simulink library "csu_ctp_coarse_thruster_pulse_command_new_lib"  (R2015b)
settings: Solver=ode113  StartTime=0.0  StopTime=10.0  RelTol=1e-3
values from neighbouring files (symbols this model uses):
  cac_acs_minimum_coarse_thruster_ontime = 30    [csc_cac_coarse_acs_ctrl_init.m]
  cac_acs_time_gain_x = 20.0    (= 20)    [csc_cac_coarse_acs_ctrl_init.m]
  cac_acs_time_gain_y = 20.0    (= 20)    [csc_cac_coarse_acs_ctrl_init.m]
  cac_acs_time_gain_z = 20.0    (= 20)    [csc_cac_coarse_acs_ctrl_init.m]
  cac_coarse_desired_thrust_gain = 1.0    (= 1)    [csc_cac_coarse_acs_ctrl_init.m]
  cac_coarse_thruster_force = psp_coarse_acs_thrust    [csc_cac_coarse_acs_ctrl_prep.m]
  cac_coarse_thruster_trq_x = cac_coarse_thruster_trq_x + cac_coarse_thruster_force*cac_coarse_trq_matx(cac_thruster_alloc_coarse_x_plus(i),1)    [csc_cac_coarse_acs_ctrl_prep.m]
  cac_coarse_thruster_trq_y = cac_coarse_thruster_trq_y + cac_coarse_thruster_force*cac_coarse_trq_matx(cac_thruster_alloc_coarse_y_plus(i),2)    [csc_cac_coarse_acs_ctrl_prep.m]
  cac_coarse_thruster_trq_z = cac_coarse_thruster_trq_z + cac_coarse_thruster_force*cac_coarse_trq_matx(cac_thruster_alloc_coarse_z_plus(i),3)    [csc_cac_coarse_acs_ctrl_prep.m]
  cac_max_thrust_to_weight_ratio = 1.05    [csc_cac_coarse_acs_ctrl_init.m]
  cac_saturation_axial_force = 0*cac_coarse_thruster_force*cosd(15)+4*cac_coarse_thruster_force    [csc_cac_coarse_acs_ctrl_prep.m]
  cac_total_trq_axial_force_matx = [cac_coarse_thruster_force*cac_coarse_trq_matx';cac_coarse_thruster_force_axial]    [csc_cac_coarse_acs_ctrl_prep.m]
undefined symbols (not defined in the file or in its folder): cac_num_variable, cac_thr_control, cac_thruster_alloc_pad_coarse_x_tq_full_on, cac_thruster_alloc_pad_coarse_x_tq_variable, cac_thruster_alloc_pad_coarse_y_tq_full_on, cac_thruster_alloc_pad_coarse_y_tq_variable, cac_trq_control, emp_initial_mass, gal_grav_surface_topo
libraries: simulink x12, util_info_lib x2
(part 2 of 2)

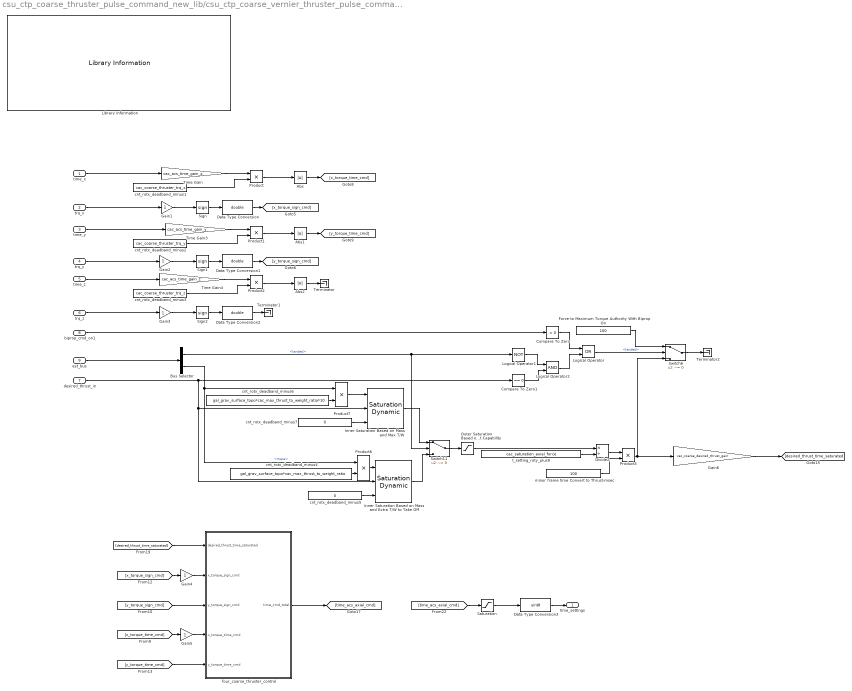
== system csu_ctp_coarse_thruster_pulse_command_new_lib/csu_ctp_coarse_vernier_thruster_pulse_command_new ==
  time_x : Inport
  "trq_x " : Inport  Port=2
  time_y : Inport  Port=3
  trq_y : Inport  Port=4
  time_z : Inport  Port=5
  trq_z : Inport  Port=6
  desired_thrust_in : Inport  Port=7
  biprop_cmd_on1 : Inport  Port=8
  est_bus : Inport  Port=9
  Abs : Abs
  Abs1 : Abs
  Abs2 : Abs
  Bus Selector : BusSelector  OutputSignals=landed,mass
  Compare To Zero : simulink/Logic and Bit Operations/Compare To Zero  relop=>  OutDataTypeStr=boolean
  Compare To Zero1 : simulink/Logic and Bit Operations/Compare To Zero  relop===  OutDataTypeStr=boolean
  Data Type Conversion : DataTypeConversion  OutDataTypeStr=double
  Data Type Conversion1 : DataTypeConversion  OutDataTypeStr=double
  Data Type Conversion2 : DataTypeConversion  OutDataTypeStr=double
  Data Type Conversion3 : DataTypeConversion  OutDataTypeStr=uint8
  Divide2 : Product  Inputs=*/
  Force to Maximum Torque Authority With Biprop On : Constant  Value=100
  Gain{1..5} (5 alike) : Gain
  Gain6 : Gain  Gain=cac_coarse_desired_thrust_gain
  Inner Saturation Based on Mass and Extra T/W to Take Off : simulink/Discontinuities/Saturation Dynamic  OutMin=[]  OutMax=[]  OutDataTypeStr=Inherit: Same as second input  OutDataType=fixdt(1, 16)  OutScaling=2^-10  DoSatur=off
  Inner Saturation Based on Mass and Max T/W : simulink/Discontinuities/Saturation Dynamic  OutMin=[]  OutMax=[]  OutDataTypeStr=Inherit: Same as second input  OutDataType=fixdt(1, 16)  OutScaling=2^-10  DoSatur=off
  Library Information : util_info_lib/Library Information  owner='NONE'
  Logical Operator : Logic  Operator=OR  AllPortsSameDT=off  OutDataTypeStr=boolean
  Logical Operator1 : Logic  Operator=NOT  AllPortsSameDT=off  OutDataTypeStr=boolean
  Logical Operator2 : Logic  AllPortsSameDT=off  OutDataTypeStr=boolean
  Outer Saturation Based on Total Thrust Capability : Saturate  UpperLimit=cac_saturation_axial_force  LowerLimit=0
  Product{,1..3,6..7} (6 alike) : Product
  Saturation : Saturate  UpperLimit=120  LowerLimit=0
  Sign : Signum
  Sign1 : Signum
  Sign2 : Signum
  Switch11 : Switch  Criteria=u2 ~= 0
  Switch6 : Switch  Criteria=u2 ~= 0
  Terminator : Terminator
  Terminator1 : Terminator
  Terminator2 : Terminator
  Time Gain : Gain  Gain=cac_acs_time_gain_x
  Time Gain3 : Gain  Gain=cac_acs_time_gain_y
  Time Gain4 : Gain  Gain=cac_acs_time_gain_z
  cnt_rotx_deadband_minus1 : Constant  Value=cac_coarse_thruster_trq_x
  cnt_rotx_deadband_minus2 : Constant  Value=cac_coarse_thruster_trq_y
  cnt_rotx_deadband_minus3 : Constant  Value=cac_coarse_thruster_trq_z
  cnt_rotx_deadband_minus4 : Constant  Value=gal_grav_surface_topo*cac_max_thrust_to_weight_ratio
  cnt_rotx_deadband_minus5 : Constant  Value=0
  cnt_rotx_deadband_minus6 : Constant  Value=gal_grav_surface_topo*cac_max_thrust_to_weight_ratio*10
  cnt_rotx_deadband_minus7 : Constant  Value=0
  four_coarse_thruster_control : MATLAB Function  TreatAsAtomicUnit=on
  "minor frame time Convert to Thrust-msec " : Constant  Value=100
  t_setting_roty_plus9 : Constant  Value=cac_saturation_axial_force
  time_settings : Outport
  wires:
  Inner Saturation Based on Mass and Max T/W/1 -> Switch11/1
  Product3/1 -> Gain6/1, Switch6/3
  Logical Operator/1 -> Switch6/2  "<landed>"
  desired_thrust_in/1 -> Inner Saturation Based on Mass and Extra T/W to Take Off/2, Inner Saturation Based on Mass and Max T/W/2, Compare To Zero1/1
  Abs1/1 -> [y_torque_time_cmd]
  Abs/1 -> [x_torque_time_cmd]
  Inner Saturation Based on Mass and Extra T/W to Take Off/1 -> Switch11/3
  Time Gain/1 -> Product/1
  Switch11/1 -> Outer Saturation Based on Total Thrust Capability/1
  Bus Selector/1 -> Switch11/2, Logical Operator1/1  "<landed>"
  Logical Operator2/1 -> Logical Operator/2
  Compare To Zero1/1 -> Logical Operator2/2
  Logical Operator1/1 -> Logical Operator2/1
  Compare To Zero/1 -> Logical Operator/1
  Force to Maximum Torque Authority With Biprop On/1 -> Switch6/1
  Outer Saturation Based on Total Thrust Capability/1 -> Divide2/1
  biprop_cmd_on1/1 -> Compare To Zero/1
  four_coarse_thruster_control/1(time_cmd_total) -> [time_acs_axial_cmd]
  Time Gain3/1 -> Product1/1
  [desired_thrust_time_saturated] -> four_coarse_thruster_control/1(desired_thrust_time_saturated)
  Time Gain4/1 -> Product2/1
  [x_torque_sign_cmd] -> Gain4/1
  Abs2/1 -> Terminator/1
  Product2/1 -> Abs2/1
  [x_torque_time_cmd] -> Gain5/1
  [y_torque_sign_cmd] -> four_coarse_thruster_control/3(y_torque_sign_cmd)
  [y_torque_time_cmd] -> four_coarse_thruster_control/5(y_torque_time_cmd)
  Data Type Conversion/1 -> [x_torque_sign_cmd]
  Data Type Conversion1/1 -> [y_torque_sign_cmd]
  Data Type Conversion2/1 -> Terminator1/1
  trq_z/1 -> Gain3/1
  Sign2/1 -> Data Type Conversion2/1
  trq_y/1 -> Gain2/1
  Sign1/1 -> Data Type Conversion1/1
  "trq_x "/1 -> Gain1/1
  Sign/1 -> Data Type Conversion/1
  Divide2/1 -> Product3/1
  t_setting_roty_plus9/1 -> Divide2/2
  "minor frame time Convert to Thrust-msec "/1 -> Product3/2
  Product1/1 -> Abs1/1
  Product/1 -> Abs/1
  cnt_rotx_deadband_minus3/1 -> Product2/2
  cnt_rotx_deadband_minus2/1 -> Product1/2
  time_z/1 -> Time Gain4/1
  time_y/1 -> Time Gain3/1
  time_x/1 -> Time Gain/1
  cnt_rotx_deadband_minus1/1 -> Product/2
  Data Type Conversion3/1 -> time_settings/1
  est_bus/1 -> Bus Selector/1
  cnt_rotx_deadband_minus5/1 -> Inner Saturation Based on Mass and Extra T/W to Take Off/3
  cnt_rotx_deadband_minus4/1 -> Product6/2
  Product6/1 -> Inner Saturation Based on Mass and Extra T/W to Take Off/1
  cnt_rotx_deadband_minus7/1 -> Inner Saturation Based on Mass and Max T/W/3
  cnt_rotx_deadband_minus6/1 -> Product7/2
  Product7/1 -> Inner Saturation Based on Mass and Max T/W/1
  Bus Selector/2 -> Product6/1, Product7/1  "<mass>"
  Gain1/1 -> Sign/1
  Gain2/1 -> Sign1/1
  Gain3/1 -> Sign2/1
  Saturation/1 -> Data Type Conversion3/1
  [time_acs_axial_cmd] -> Saturation/1
  Switch6/1 -> Terminator2/1
  Gain4/1 -> four_coarse_thruster_control/2(x_torque_sign_cmd)
  Gain5/1 -> four_coarse_thruster_control/4(x_torque_time_cmd)
  Gain6/1 -> [desired_thrust_time_saturated]

== matlab function csu_ctp_coarse_thruster_pulse_command_new_lib/csu_ctp_coarse_thruster_pulse_command_short_fire/MATLAB Function ==
  data: x_torque_sign_cmd input; y_torque_sign_cmd input; z_torque_sign_cmd input; x_torque_time_cmd input; y_torque_time_cmd input; z_torque_time_cmd input; x_sorted_thrust_cmd input; y_sorted_thrust_cmd input; desired_thrust_saturated input; cac_trq_control input; cac_thr_control input; cac_thruster_alloc_pad_coarse_x_tq_full_on input; cac_thruster_alloc_pad_coarse_y_tq_full_on input; cac_thruster_alloc_pad_coarse_x_tq_variable input; cac_thruster_alloc_pad_coarse_y_tq_variable input; cac_num_variable input; cac_total_trq_axial_force_matx input; cac_coarse_thruster_trq_x input; cac_coarse_thruster_trq_y input; cac_coarse_thruster_trq_z input; cac_saturation_axial_force input; time_cmd_total output; max_offset_x output; max_offset_y output; dist_thrust_x output; dist_thrust_y output; zone_radius output; radius_minus_distance_x output; radius_minus_distance_y output; imax_x output; imax_y output; delta_thr_x output; delta_thr_y output; delta_trq_x output; delta_trq_y output; coarse_tq_full_on_x output; coarse_tq_full_on_y output; time_axial_cmd output; torq_axial_cmd output; cac_trq_axial_force_pinv_reduced_matx output
function [time_cmd_total,max_offset_x,max_offset_y,...
    dist_thrust_x,dist_thrust_y,...
    zone_radius,...
    radius_minus_distance_x,radius_minus_distance_y,...
    imax_x,imax_y,...
    delta_thr_x,delta_thr_y,...
    delta_trq_x,delta_trq_y,...
    coarse_tq_full_on_x,coarse_tq_full_on_y,...
    time_axial_cmd,torq_axial_cmd,...
    cac_trq_axial_force_pinv_reduced_matx...
     ]...
     =...
                         find_thruster_combination(...
                         x_torque_sign_cmd,...
                         y_torque_sign_cmd,...
                         z_torque_sign_cmd,...
                         x_torque_time_cmd,...
                         y_torque_time_cmd,...
                         z_torque_time_cmd,...
                         x_sorted_thrust_cmd,...
                         y_sorted_thrust_cmd,...
                         desired_thrust_saturated,...
                         cac_trq_control,...
                         cac_thr_control,...
                         cac_thruster_alloc_pad_coarse_x_tq_full_on,...
                         cac_thruster_alloc_pad_coarse_y_tq_full_on,...
                         cac_thruster_alloc_pad_coarse_x_tq_variable,...
                         cac_thruster_alloc_pad_coarse_y_tq_variable,...
                         cac_num_variable,...
                         cac_total_trq_axial_force_matx,...
                         cac_coarse_thruster_trq_x,...
                         cac_coarse_thruster_trq_y,...
                         cac_coarse_thruster_trq_z,...
                         cac_saturation_axial_force...
                         )         
%#codegen

delta_thr_x = zeros(21,1);
delta_thr_y = zeros(21,1);
delta_trq_x = zeros(21,1);
delta_trq_y = zeros(21,1);
dist_thrust_x = zeros(21,1);
dist_thrust_y = zeros(21,1);
zone_radius = zeros(21,1);
radius_minus_distance_x = zeros(21,1);
radius_minus_distance_y = zeros(21,1);
cac_trq_axial_force_reduced_matx = zeros(4,12);

for i=1:size(cac_thr_control,1);
    delta_thr_x(i) = abs(cac_thr_control(i) - x_sorted_thrust_cmd);
    delta_thr_y(i) = abs(cac_thr_control(i) - y_sorted_thrust_cmd);
    
    delta_trq_x(i) = abs(x_torque_sign_cmd*x_torque_time_cmd - cac_trq_control(i));
    delta_trq_y(i) = abs(y_torque_sign_cmd*y_torque_time_cmd - cac_trq_control(i));
    
    dist_thrust_x(i) = sqrt(delta_thr_x(i)^2 + delta_trq_x(i)^2);
    dist_thrust_y(i) = sqrt(delta_thr_y(i)^2 + delta_trq_y(i)^2);
    
    zone_radius(i) = 25 * cac_num_variable(i) * sqrt(2)/2;
    
    radius_minus_distance_x(i) = zone_radius(i) - dist_thrust_x(i);
    radius_minus_distance_y(i) = zone_radius(i) - dist_thrust_y(i);
    
end

[x,imax_x] = max(radius_minus_distance_x);
[y,imax_y] = max(radius_minus_distance_y);
max_offset_x = max(radius_minus_distance_x);
max_offset_y = max(radius_minus_distance_y);

coarse_tq_full_on_x = cac_thruster_alloc_pad_coarse_x_tq_full_on(imax_x,:);
coarse_tq_full_on_y = cac_thruster_alloc_pad_coarse_y_tq_full_on(imax_y,:);

coarse_tq_variable_on_x = cac_thruster_alloc_pad_coarse_x_tq_variable(imax_x,:);
coarse_tq_variable_on_y = cac_thruster_alloc_pad_coarse_y_tq_variable(imax_y,:);

% if max_offset_x <= 0
%     coarse_tq_full_on_x = coarse_tq_full_on_x*0;
%     coarse_tq_variable_on_x = coarse_tq_variable_on_x*0;
% end
% if max_offset_x <= 0
%     coarse_tq_full_on_y = coarse_tq_full_on_y*0;
%     coarse_tq_variable_on_y = coarse_tq_variable_on_y*0;    
% end
% 
for i=1:size(cac_total_trq_axial_force_matx,1)
    cac_trq_axial_force_reduced_matx(i,:) = (cac_total_trq_axial_force_matx(i,:).*(coarse_tq_variable_on_x + coarse_tq_variable_on_y));
end    
cac_trq_axial_force_pinv_reduced_matx = pinv(cac_trq_axial_force_reduced_matx);

time_x_tq_cmd = cac_coarse_thruster_trq_x * x_torque_time_cmd * x_torque_sign_cmd;
time_y_tq_cmd = cac_coarse_thruster_trq_y * y_torque_time_cmd * y_torque_sign_cmd;
time_z_tq_cmd = cac_coarse_thruster_trq_z * z_torque_time_cmd * z_torque_sign_cmd;

time_axial_cmd = 0.0;

if(desired_thrust_saturated > 0.001)
    time_axial_cmd = (x_sorted_thrust_cmd + y_sorted_thrust_cmd)*50;%*desired_thrust_saturated;%*sum(coarse_tq_variable_on_x + coarse_tq_variable_on_y);
end

torq_axial_cmd = [time_x_tq_cmd; time_y_tq_cmd; time_z_tq_cmd ; time_axial_cmd];
time_cmd_total = cac_trq_axial_force_pinv_reduced_matx*torq_axial_cmd + (coarse_tq_full_on_x + coarse_tq_full_on_y)'*100;

== matlab function csu_ctp_coarse_thruster_pulse_command_new_lib/csu_ctp_coarse_thruster_pulse_command_old/MATLAB Function ==
  data: x_torque_sign_cmd input; y_torque_sign_cmd input; z_torque_sign_cmd input; x_torque_time_cmd input; y_torque_time_cmd input; z_torque_time_cmd input; x_sorted_thrust_cmd input; y_sorted_thrust_cmd input; desired_thrust_saturated input; cac_trq_control input; cac_thr_control input; cac_thruster_alloc_pad_coarse_x_tq_full_on input; cac_thruster_alloc_pad_coarse_y_tq_full_on input; cac_thruster_alloc_pad_coarse_x_tq_variable input; cac_thruster_alloc_pad_coarse_y_tq_variable input; cac_num_variable input; cac_total_trq_axial_force_matx input; cac_coarse_thruster_trq_x input; cac_coarse_thruster_trq_y input; cac_coarse_thruster_trq_z input; cac_saturation_axial_force input; time_cmd_total output; max_offset_x output; max_offset_y output; dist_thrust_x output; dist_thrust_y output; zone_radius output; radius_minus_distance_x output; radius_minus_distance_y output; imax_x output; imax_y output; delta_thr_x output; delta_thr_y output; delta_trq_x output; delta_trq_y output; coarse_tq_full_on_x output; coarse_tq_full_on_y output; time_axial_cmd output; torq_axial_cmd output; cac_trq_axial_force_pinv_reduced_matx output
function [time_cmd_total,max_offset_x,max_offset_y,...
    dist_thrust_x,dist_thrust_y,...
    zone_radius,...
    radius_minus_distance_x,radius_minus_distance_y,...
    imax_x,imax_y,...
    delta_thr_x,delta_thr_y,...
    delta_trq_x,delta_trq_y,...
    coarse_tq_full_on_x,coarse_tq_full_on_y,...
    time_axial_cmd,torq_axial_cmd,...
    cac_trq_axial_force_pinv_reduced_matx...
     ]...
     =...
                         find_thruster_combination(...
                         x_torque_sign_cmd,...
                         y_torque_sign_cmd,...
                         z_torque_sign_cmd,...
                         x_torque_time_cmd,...
                         y_torque_time_cmd,...
                         z_torque_time_cmd,...
                         x_sorted_thrust_cmd,...
                         y_sorted_thrust_cmd,...
                         desired_thrust_saturated,...
                         cac_trq_control,...
                         cac_thr_control,...
                         cac_thruster_alloc_pad_coarse_x_tq_full_on,...
                         cac_thruster_alloc_pad_coarse_y_tq_full_on,...
                         cac_thruster_alloc_pad_coarse_x_tq_variable,...
                         cac_thruster_alloc_pad_coarse_y_tq_variable,...
                         cac_num_variable,...
                         cac_total_trq_axial_force_matx,...
                         cac_coarse_thruster_trq_x,...
                         cac_coarse_thruster_trq_y,...
                         cac_coarse_thruster_trq_z,...
                         cac_saturation_axial_force...
                         )         
%#codegen

delta_thr_x = zeros(21,1);
delta_thr_y = zeros(21,1);
delta_trq_x = zeros(21,1);
delta_trq_y = zeros(21,1);
dist_thrust_x = zeros(21,1);
dist_thrust_y = zeros(21,1);
zone_radius = zeros(21,1);
radius_minus_distance_x = zeros(21,1);
radius_minus_distance_y = zeros(21,1);
cac_trq_axial_force_reduced_matx = zeros(4,12);

for i=1:size(cac_thr_control,1);
    delta_thr_x(i) = abs(cac_thr_control(i) - x_sorted_thrust_cmd);
    delta_thr_y(i) = abs(cac_thr_control(i) - y_sorted_thrust_cmd);
    
    delta_trq_x(i) = abs(x_torque_sign_cmd*x_torque_time_cmd - cac_trq_control(i));
    delta_trq_y(i) = abs(y_torque_sign_cmd*y_torque_time_cmd - cac_trq_control(i));
    
    dist_thrust_x(i) = sqrt(delta_thr_x(i)^2 + delta_trq_x(i)^2);
    dist_thrust_y(i) = sqrt(delta_thr_y(i)^2 + delta_trq_y(i)^2);
    
    zone_radius(i) = 25 * cac_num_variable(i) * sqrt(2)/2;
    
    radius_minus_distance_x(i) = zone_radius(i) - dist_thrust_x(i);
    radius_minus_distance_y(i) = zone_radius(i) - dist_thrust_y(i);
    
end

[x,imax_x] = max(radius_minus_distance_x);
[y,imax_y] = max(radius_minus_distance_y);
max_offset_x = max(radius_minus_distance_x);
max_offset_y = max(radius_minus_distance_y);

coarse_tq_full_on_x = cac_thruster_alloc_pad_coarse_x_tq_full_on(imax_x,:);
coarse_tq_full_on_y = cac_thruster_alloc_pad_coarse_y_tq_full_on(imax_y,:);

coarse_tq_variable_on_x = cac_thruster_alloc_pad_coarse_x_tq_variable(imax_x,:);
coarse_tq_variable_on_y = cac_thruster_alloc_pad_coarse_y_tq_variable(imax_y,:);

% if max_offset_x <= 0
%     coarse_tq_full_on_x = coarse_tq_full_on_x*0;
%     coarse_tq_variable_on_x = coarse_tq_variable_on_x*0;
% end
% if max_offset_x <= 0
%     coarse_tq_full_on_y = coarse_tq_full_on_y*0;
%     coarse_tq_variable_on_y = coarse_tq_variable_on_y*0;    
% end
% 
for i=1:size(cac_total_trq_axial_force_matx,1)
    cac_trq_axial_force_reduced_matx(i,:) = (cac_total_trq_axial_force_matx(i,:).*(coarse_tq_variable_on_x + coarse_tq_variable_on_y));
end    
cac_trq_axial_force_pinv_reduced_matx = pinv(cac_trq_axial_force_reduced_matx);

time_x_tq_cmd = cac_coarse_thruster_trq_x * x_torque_time_cmd * x_torque_sign_cmd;
time_y_tq_cmd = cac_coarse_thruster_trq_y * y_torque_time_cmd * y_torque_sign_cmd;
time_z_tq_cmd = cac_coarse_thruster_trq_z * z_torque_time_cmd * z_torque_sign_cmd;

time_axial_cmd = 0.0;

if(desired_thrust_saturated > 0.001)
    time_axial_cmd = (x_sorted_thrust_cmd + y_sorted_thrust_cmd)*50;%*desired_thrust_saturated;%*sum(coarse_tq_variable_on_x + coarse_tq_variable_on_y);
end

torq_axial_cmd = [time_x_tq_cmd; time_y_tq_cmd; time_z_tq_cmd ; time_axial_cmd];
time_cmd_total = cac_trq_axial_force_pinv_reduced_matx*torq_axial_cmd + (coarse_tq_full_on_x + coarse_tq_full_on_y)'*100;

== matlab function csu_ctp_coarse_thruster_pulse_command_new_lib/csu_ctp_coarse_thruster_pulse_command_new/MATLAB Function ==
  data: x_torque_sign_cmd input; y_torque_sign_cmd input; z_torque_sign_cmd input; x_torque_time_cmd input; y_torque_time_cmd input; z_torque_time_cmd input; x_sorted_thrust_cmd input; y_sorted_thrust_cmd input; desired_thrust_saturated input; cac_trq_control input; cac_thr_control input; cac_thruster_alloc_pad_coarse_x_tq_full_on input; cac_thruster_alloc_pad_coarse_y_tq_full_on input; cac_thruster_alloc_pad_coarse_x_tq_variable input; cac_thruster_alloc_pad_coarse_y_tq_variable input; cac_num_variable input; cac_total_trq_axial_force_matx input; cac_coarse_thruster_trq_x input; cac_coarse_thruster_trq_y input; cac_coarse_thruster_trq_z input; cac_saturation_axial_force input; time_cmd_total output; max_offset_x output; max_offset_y output; dist_thrust_x output; dist_thrust_y output; zone_radius output; radius_minus_distance_x output; radius_minus_distance_y output; imax_x output; imax_y output; delta_thr_x output; delta_thr_y output; delta_trq_x output; delta_trq_y output; coarse_tq_full_on_x output; coarse_tq_full_on_y output; time_axial_cmd output; torq_axial_cmd output; cac_trq_axial_force_pinv_reduced_matx output
function [time_cmd_total,max_offset_x,max_offset_y,...
    dist_thrust_x,dist_thrust_y,...
    zone_radius,...
    radius_minus_distance_x,radius_minus_distance_y,...
    imax_x,imax_y,...
    delta_thr_x,delta_thr_y,...
    delta_trq_x,delta_trq_y,...
    coarse_tq_full_on_x,coarse_tq_full_on_y,...
    time_axial_cmd,torq_axial_cmd,...
    cac_trq_axial_force_pinv_reduced_matx...
     ]...
     =...
                         find_thruster_combination(...
                         x_torque_sign_cmd,...
                         y_torque_sign_cmd,...
                         z_torque_sign_cmd,...
                         x_torque_time_cmd,...
                         y_torque_time_cmd,...
                         z_torque_time_cmd,...
                         x_sorted_thrust_cmd,...
                         y_sorted_thrust_cmd,...
                         desired_thrust_saturated,...
                         cac_trq_control,...
                         cac_thr_control,...
                         cac_thruster_alloc_pad_coarse_x_tq_full_on,...
                         cac_thruster_alloc_pad_coarse_y_tq_full_on,...
                         cac_thruster_alloc_pad_coarse_x_tq_variable,...
                         cac_thruster_alloc_pad_coarse_y_tq_variable,...
                         cac_num_variable,...
                         cac_total_trq_axial_force_matx,...
                         cac_coarse_thruster_trq_x,...
                         cac_coarse_thruster_trq_y,...
                         cac_coarse_thruster_trq_z,...
                         cac_saturation_axial_force...
                         )         
%#codegen

delta_thr_x = zeros(21,1);
delta_thr_y = zeros(21,1);
delta_trq_x = zeros(21,1);
delta_trq_y = zeros(21,1);
dist_thrust_x = zeros(21,1);
dist_thrust_y = zeros(21,1);
zone_radius = zeros(21,1);
radius_minus_distance_x = zeros(21,1);
radius_minus_distance_y = zeros(21,1);
cac_trq_axial_force_reduced_matx = zeros(4,12);

for i=1:size(cac_thr_control,1);
    delta_thr_x(i) = abs(cac_thr_control(i) - x_sorted_thrust_cmd);
    delta_thr_y(i) = abs(cac_thr_control(i) - y_sorted_thrust_cmd);
    
    delta_trq_x(i) = abs(x_torque_sign_cmd*x_torque_time_cmd - cac_trq_control(i));
    delta_trq_y(i) = abs(y_torque_sign_cmd*y_torque_time_cmd - cac_trq_control(i));
    
    dist_thrust_x(i) = sqrt(delta_thr_x(i)^2 + delta_trq_x(i)^2);
    dist_thrust_y(i) = sqrt(delta_thr_y(i)^2 + delta_trq_y(i)^2);
    
    zone_radius(i) = 25 * cac_num_variable(i) * sqrt(2)/2;
    
    radius_minus_distance_x(i) = zone_radius(i) - dist_thrust_x(i);
    radius_minus_distance_y(i) = zone_radius(i) - dist_thrust_y(i);
    
end

[x,imax_x] = max(radius_minus_distance_x);
[y,imax_y] = max(radius_minus_distance_y);
max_offset_x = max(radius_minus_distance_x);
max_offset_y = max(radius_minus_distance_y);

coarse_tq_full_on_x = cac_thruster_alloc_pad_coarse_x_tq_full_on(imax_x,:);
coarse_tq_full_on_y = cac_thruster_alloc_pad_coarse_y_tq_full_on(imax_y,:);

coarse_tq_variable_on_x = cac_thruster_alloc_pad_coarse_x_tq_variable(imax_x,:);
coarse_tq_variable_on_y = cac_thruster_alloc_pad_coarse_y_tq_variable(imax_y,:);

% if max_offset_x <= 0
%     coarse_tq_full_on_x = coarse_tq_full_on_x*0;
%     coarse_tq_variable_on_x = coarse_tq_variable_on_x*0;
% end
% if max_offset_x <= 0
%     coarse_tq_full_on_y = coarse_tq_full_on_y*0;
%     coarse_tq_variable_on_y = coarse_tq_variable_on_y*0;    
% end
% 
for i=1:size(cac_total_trq_axial_force_matx,1)
    cac_trq_axial_force_reduced_matx(i,:) = (cac_total_trq_axial_force_matx(i,:).*(coarse_tq_variable_on_x + coarse_tq_variable_on_y));
end    
cac_trq_axial_force_pinv_reduced_matx = pinv(cac_trq_axial_force_reduced_matx);

time_x_tq_cmd = cac_coarse_thruster_trq_x * x_torque_time_cmd * x_torque_sign_cmd;
time_y_tq_cmd = cac_coarse_thruster_trq_y * y_torque_time_cmd * y_torque_sign_cmd;
time_z_tq_cmd = cac_coarse_thruster_trq_z * z_torque_time_cmd * z_torque_sign_cmd;

time_axial_cmd = 0.0;

if(desired_thrust_saturated > 0.001)
    time_axial_cmd = (x_sorted_thrust_cmd + y_sorted_thrust_cmd)*50;%*desired_thrust_saturated;%*sum(coarse_tq_variable_on_x + coarse_tq_variable_on_y);
end

torq_axial_cmd = [time_x_tq_cmd; time_y_tq_cmd; time_z_tq_cmd ; time_axial_cmd];
time_cmd_total = cac_trq_axial_force_pinv_reduced_matx*torq_axial_cmd + (coarse_tq_full_on_x + coarse_tq_full_on_y)'*100;

== matlab function csu_ctp_coarse_thruster_pulse_command_new_lib/csu_ctp_coarse_vernier_thruster_pulse_command_new/four_coarse_thruster_control ==
  data: desired_thrust_time_saturated input; x_torque_sign_cmd input; y_torque_sign_cmd input; x_torque_time_cmd input; y_torque_time_cmd input; time_cmd_total output
function time_cmd_total  = four_coarse_thruster_control(...
                             desired_thrust_time_saturated,...
                             x_torque_sign_cmd,...
                             y_torque_sign_cmd,...
                             x_torque_time_cmd,...
                             y_torque_time_cmd)...         
%#codegen

time_cmd_total = [0 0 0 0 0 0 0 0 0 0 0 0]';

if desired_thrust_time_saturated > 0
    
    time_cmd_total(2) =  desired_thrust_time_saturated;
    time_cmd_total(5) =  desired_thrust_time_saturated;
    time_cmd_total(8) =  desired_thrust_time_saturated;
    time_cmd_total(11) = desired_thrust_time_saturated;

    if x_torque_sign_cmd < 0
        if x_torque_time_cmd >= desired_thrust_time_saturated
            time_cmd_total(5) = x_torque_time_cmd - desired_thrust_time_saturated
        else
            time_cmd_total(5) = desired_thrust_time_saturated - x_torque_time_cmd
        end
    end
    if x_torque_sign_cmd > 0
        if x_torque_time_cmd >= desired_thrust_time_saturated
            time_cmd_total(11) = x_torque_time_cmd - desired_thrust_time_saturated;
        else
            time_cmd_total(11) = desired_thrust_time_saturated - x_torque_time_cmd;
        end
    end
    
    if y_torque_sign_cmd < 0
        if y_torque_time_cmd >= desired_thrust_time_saturated
            time_cmd_total(8) = y_torque_time_cmd - desired_thrust_time_saturated;
        else
            time_cmd_total(8) = desired_thrust_time_saturated - y_torque_time_cmd;
        end
    end
    if y_torque_sign_cmd > 0
        if y_torque_time_cmd >= desired_thrust_time_saturated
            time_cmd_total(2) = y_torque_time_cmd - desired_thrust_time_saturated;
        else
            time_cmd_total(2) = desired_thrust_time_saturated - y_torque_time_cmd;
        end
    end
    
else
    
    if x_torque_sign_cmd < 0
        time_cmd_total(11) = x_torque_time_cmd;
    elseif x_torque_sign_cmd > 0
        time_cmd_total(5) = x_torque_time_cmd
    end
    
    if y_torque_sign_cmd < 0
        time_cmd_total(2) = y_torque_time_cmd;
    elseif y_torque_sign_cmd > 0
        time_cmd_total(8) = y_torque_time_cmd;
    end
end
